simulink model "linearAircraft"  (R2023b)
settings: Solver=VariableStepAuto  StartTime=0.0  StopTime=10.0  RelTol=1e-3
undefined symbols (not defined in the file or in its folder): lat, lon
libraries: cstblocks x2
settings Model: Creator=Victor  LastModifiedBy=Victor

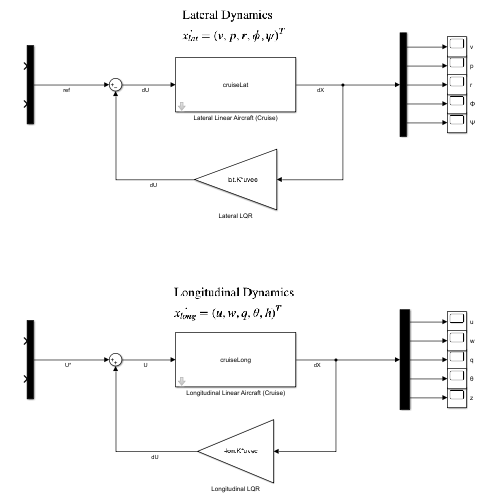
[thumbnail: Simulink's stored preview of the top-level diagram]
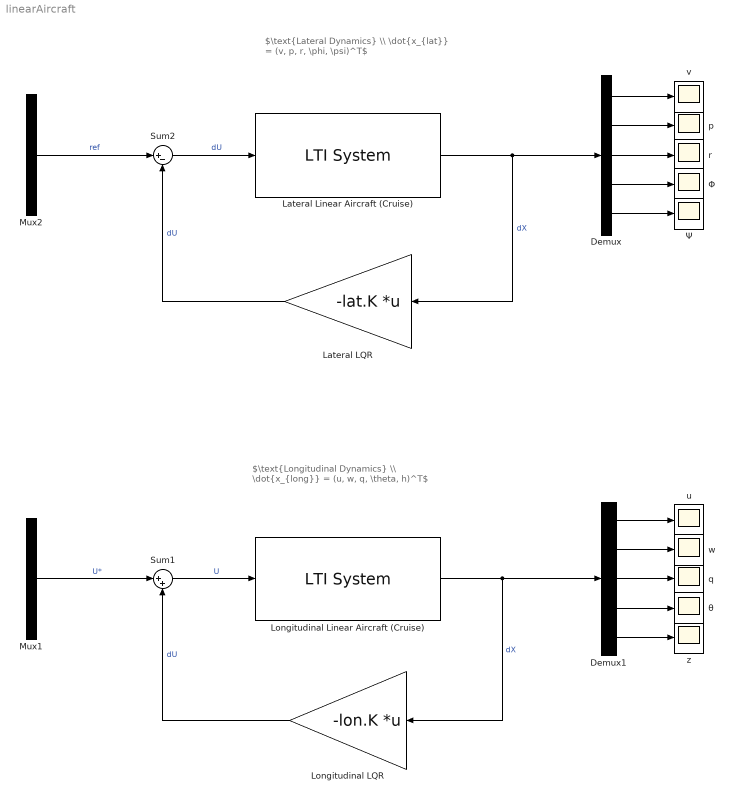
== system linearAircraft ==
  note: $\text{Lateral Dynamics} \\ \dot{x_{lat}} = (v, p, r, \phi, \psi)^T$
  note: $\text{Longitudinal Dynamics} \\ \dot{x_{long}} = (u, w, q, \theta, h)^T$
  Demux : Demux  Outputs=5
  Demux1 : Demux  Outputs=5
  Lateral LQR : Gain  Gain=-lat.K  Multiplication=Matrix(K*u) (u vector)
  Lateral Linear Aircraft (Cruise) : cstblocks/LTI System  sys=cruiseLat  IC=[lat.theta0, lat.w0, lat.v0]  PadeOrder=0
  Longitudinal LQR : Gain  Gain=-lon.K  Multiplication=Matrix(K*u) (u vector)
  Longitudinal Linear Aircraft (Cruise) : cstblocks/LTI System  sys=cruiseLong  IC=[lon.theta0, lon.w0, lon.v0, lon.x0]  PadeOrder=0
  Mux1 : Mux  Inputs=2
  Mux2 : Mux  Inputs=2
  Sum1 : Sum  Inputs=|++
  Sum2 : Sum  Inputs=|+-
  p : Scope
  q : Scope
  r : Scope
  u : Scope
  v : Scope
  w : Scope
  z : Scope
  Φ : Scope
  Ψ : Scope
  θ : Scope
  wires:
  Lateral Linear Aircraft (Cruise)/1 -> Lateral LQR/1, Demux/1  "dX"
  Longitudinal Linear Aircraft (Cruise)/1 -> Longitudinal LQR/1, Demux1/1  "dX"
  Demux/1 -> v/1
  Demux/2 -> p/1
  Demux/3 -> r/1
  Demux/4 -> Φ/1
  Demux/5 -> Ψ/1
  Demux1/1 -> u/1
  Demux1/2 -> w/1
  Demux1/3 -> q/1
  Demux1/4 -> θ/1
  Demux1/5 -> z/1
  Lateral LQR/1 -> Sum2/2  "dU"
  Sum2/1 -> Lateral Linear Aircraft (Cruise)/1  "dU"
  Mux2/1 -> Sum2/1  "ref"
  Mux1/1 -> Sum1/1  "U*"
  Sum1/1 -> Longitudinal Linear Aircraft (Cruise)/1  "U"
  Longitudinal LQR/1 -> Sum1/2  "dU"
